simulink model "vipstripes"  (R2017b)
settings: Solver=FixedStepDiscrete  StartTime=0.0  StopTime=inf  RelTol=1e-3  EnableMultiTasking=on
model workspace (MATLAB code in the model file):
  | % Define image size and padded size.
  | imgSize = [120 160];
  | paddedSize = 2^ceil(log2(max(imgSize)));
  | 
  | % Load and initialize the data required by vipstripes demo.
  | cf = 0.65;
  | f = cf-0.04:0.005:cf+0.04;
  | f = repmat(f,[7,1]);
  | f = f(:);
  | ft.time=[];
  | ft.signals.values=f;
  | ft.signals.dimensions=1;
  | p = 0:0.5:3;
  | pt.time=[];
  | pt.signals.values=p';
  | pt.signals.dimensions= 1;
  | % FIR least-squares Bandstop filter designed using the FIRLS function.
  | % dfilt requires Signal Processing Toolbox license
  | % All frequency values are normalized to 1.
  | % N      = 30;    % Order
  | % Fpass1 = 0.51;  % First Passband Frequency
  | % Fstop1 = 0.6;   % First Stopband Frequency
  | % Fstop2 = 0.7;   % Second Stopband Frequency
  | % Fpass2 = 0.79;  % Second Passband Frequency
  | % Wpass1 = 1;     % First Passband Weight
  | % Wstop  = 1;     % Stopband Weight
  | % Wpass2 = 1;     % Second Passband Weight
  | % % Calculate the coefficients using the FIRLS function.
  | % Hd = dfilt.dffir(firls(N, [0 Fpass1 Fstop1 Fstop2 Fpass2 1], ...
  | %            [1 1 0 0 1 1], [Wpass1 Wstop Wpass2]));
  | %
  | % % Extract filter coefficients from the filter object
  | % b  = Hd.Numerator;
  | b = [ 0.0128   -0.0172    0.0010    0.0153   -0.0098 ...
  |       0.0002   -0.0149    0.0283    0.0129   -0.0852 ...
  |       0.0790    0.0478   -0.1639    0.1058    0.0897 ...
  |       0.8012    0.0897    0.1058   -0.1639    0.0478 ...
  |       0.0790   -0.0852    0.0129    0.0283   -0.0149 ...
  |       0.0002   -0.0098    0.0153    0.0010   -0.0172 ...
  |       0.0128 ];
  | % Convert the one-dimensional filter to 2-D using ftrans2 function from
  | % the Image Processing toolbox
  | h = ftrans2(b);
undefined symbols (not defined in the file or in its folder): gray
libraries: visiontransforms x2, visiontextngfix x2, visiongeotforms x2, visionutilities x1, visionfilter x1, vipmisc x1, dspvision x1
settings Model: FPTRunName=Active  ExtModeAutoUpdateStatusClock=off  Creator=The MathWorks, Inc.  LastModifiedBy=The MathWorks, Inc.
settings DataIOCC: LimitDataPoints=on  SaveFormat=Array  SaveOutput=off  SaveTime=off  SignalLoggingName=logsOut
settings OptimizationCC: ExpressionDepthLimit=2147483647  InitFltsAndDblsToZero=on  EfficientMapNaN2IntZero=off  LifeSpan=inf
settings DebuggingCC: SaveWithParameterizedLinksMsg=none  UnderspecifiedInitializationDetection=Classic  MergeDetectMultiDrivingBlocksExec=none  CheckExecutionContextPreStartOutputMsg=on  CheckExecutionContextRuntimeOutputMsg=on  SignalResolutionControl=TryResolveAllWithWarning  InheritedTsInSrcMsg=none  MultiTaskDSMMsg=warning  MultiTaskCondExecSysMsg=none  SigSpecEnsureSampleTimeMsg=none  ParameterPrecisionLossMsg=none  FcnCallInpInsideContextMsg=warning  AllowSymbolicDim=off  StateNameClashWarn=warning  SFUnexpectedBacktrackingDiag=warning  SFNoUnconditionalDefaultTransitionDiag=warning  SFExecutionAtInitializationDiag=none
settings HardwareCC: ProdBitPerPointer=32  ProdBitPerSizeT=32  ProdBitPerPtrDiffT=32  ProdLargestAtomicFloat=None  ProdIntDivRoundTo=Undefined  ProdEndianess=Unspecified  ProdWordSize=32  ProdHWDeviceType=32-bit Generic  TargetBitPerPointer=64  TargetBitPerSizeT=64  TargetBitPerPtrDiffT=64  TargetLongLongMode=on  TargetIntDivRoundTo=Zero  TargetEndianess=LittleEndian  TargetWordSize=64  TargetHWDeviceType=Generic->MATLAB Host Computer  ProdEqTarget=off
settings ModelReferenceCC: PropagateSignalLabelsOutOfModel=off
settings CodeAppCC: StateflowObjectComments=on
settings GRTTargetCC: TargetFcnLib=ansi_tfl_tmw.mat  TargetLangStandard=C89/C90 (ANSI)  GeneratePreprocessorConditionals=Disable all  CombineOutputUpdateFcns=off  GRTInterface=on
settings ConfigComp: CovMetricSettings=dw  CovHtmlReporting=on  CovSaveCumulativeToWorkspaceVar=on  CovSaveSingleToWorkspaceVar=on  CovExternalEMLEnable=off

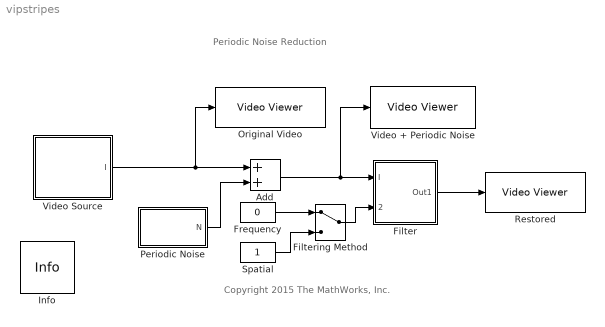
== system vipstripes ==
  note: Periodic Noise Reduction
  note: Copyright 2015 The MathWorks, Inc.
  Add : Sum
  Filter : Subsystem
  Filtering Method : ManualSwitch
  Frequency : Constant  Value=0
  Info : vipmisc/Info  SystemSampleTime=-1
      settings: SourceProductName=Computer Vision System Toolbox  SourceProductBaseCode=VP
  Original Video : VideoViewer  colormapValue=gray(256)  FigPos=[53 238 172 137]  trueSizedOnce=on
  Periodic Noise : Subsystem
  Restored : VideoViewer  colormapValue=gray(256)  FigPos=[50 623 172 127]  trueSizedOnce=on
  "Spatial " : Constant
  Video + Periodic Noise : VideoViewer  colormapValue=gray(256)  FigPos=[52 430 172 126]  trueSizedOnce=on
  Video Source : Subsystem
  wires:
  Video Source/1(I) -> Add/1, Original Video/1
  Periodic Noise/1(N) -> Add/2
  Add/1 -> Filter/1(I), Video + Periodic Noise/1
  Filter/1(Out1) -> Restored/1
  Frequency/1 -> Filtering Method/1
  "Spatial "/1 -> Filtering Method/2
  Filtering Method/1 -> Filter/2(Method)

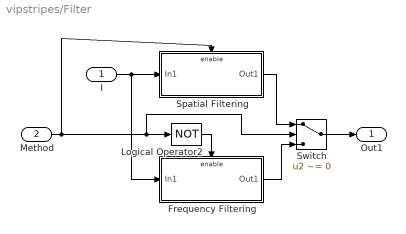
== system vipstripes/Filter ==
  I : Inport
  Method : Inport  Port=2
  Frequency Filtering : Subsystem  TreatAsAtomicUnit=on
  Logical Operator2 : Logic  Operator=NOT  AllPortsSameDT=off  OutDataTypeStr=boolean
  Spatial Filtering : Subsystem  TreatAsAtomicUnit=on
  Switch : Switch  Criteria=u2 ~= 0  ZeroCross=off
  Out1 : Outport
  wires:
  Logical Operator2/1 -> Frequency Filtering/Enable
  Method/1 -> Switch/2, Logical Operator2/1, Spatial Filtering/Enable
  Switch/1 -> Out1/1
  Frequency Filtering/1(Out1) -> Switch/3
  Spatial Filtering/1(Out1) -> Switch/1
  I/1 -> Frequency Filtering/1(In1), Spatial Filtering/1(In1)

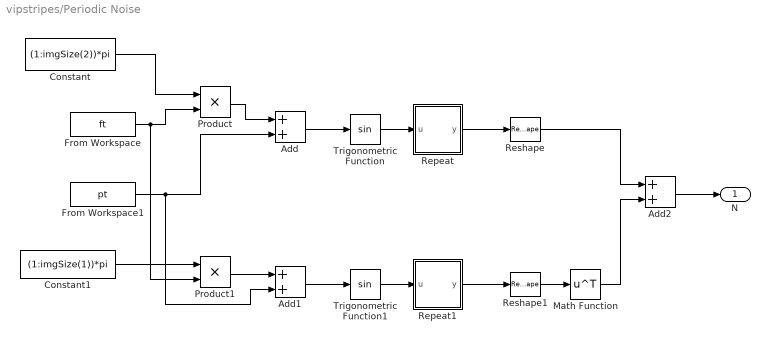
== system vipstripes/Periodic Noise ==
  Add : Sum
  Add1 : Sum
  Add2 : Sum
  Constant : Constant  Value=(1:imgSize(2))*pi
  Constant1 : Constant  Value=(1:imgSize(1))*pi
  From Workspace : FromWorkspace  VariableName=ft  Interpolate=off  OutputAfterFinalValue=Cyclic repetition
  From Workspace1 : FromWorkspace  VariableName=pt  Interpolate=off  OutputAfterFinalValue=Cyclic repetition
  Math Function : Math  Operator=transpose  SaturateOnIntegerOverflow=on
  Product : Product  RndMeth=Zero
  Product1 : Product  RndMeth=Zero
  Repeat : MATLAB Function  TreatAsAtomicUnit=on
  Repeat1 : MATLAB Function  TreatAsAtomicUnit=on
  Reshape : Reshape  OutputDimensionality=Customize  OutputDimensions=imgSize
  Reshape1 : Reshape  OutputDimensionality=Customize  OutputDimensions=fliplr(imgSize)
  Trigonometric Function : Trigonometry
  Trigonometric Function1 : Trigonometry
  N : Outport
  wires:
  Constant/1 -> Product/1
  From Workspace/1 -> Product/2, Product1/2
  Product/1 -> Add/1
  From Workspace1/1 -> Add/2, Add1/2
  Add/1 -> Trigonometric Function/1
  Trigonometric Function/1 -> Repeat/1(u)
  Repeat/1(y) -> Reshape/1
  Reshape/1 -> Add2/1
  Constant1/1 -> Product1/1
  Product1/1 -> Add1/1
  Add1/1 -> Trigonometric Function1/1
  Trigonometric Function1/1 -> Repeat1/1(u)
  Repeat1/1(y) -> Reshape1/1
  Reshape1/1 -> Math Function/1
  Math Function/1 -> Add2/2
  Add2/1 -> N/1

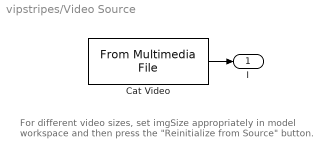
== system vipstripes/Video Source ==
  note: For different video sizes, set imgSize appropriately in model
      | workspace and then press the "Reinitialize from Source" button.
  Cat Video : dspvision/From Multimedia File  inputFilename=viptraffic.avi  loop=on  numPlays=inf  outputStreams=Video only  videoDataType=double  audioDataType=int16  inheritSampleTime=on  userDefinedSampleTime=1/30  noAudioOutput=off  isIntensityVideo=off  fourcc=Intensity  colorVideoFormat=Separate color signals  outputEOF=off  dataOrg=Column-major  audioFrameSize=1024  computeAudioFrameSize=off  outSamplingMode=Frame based
      settings: SourceProductBaseCode=VP
  I : Outport
  wires:
  Cat Video/1 -> I/1

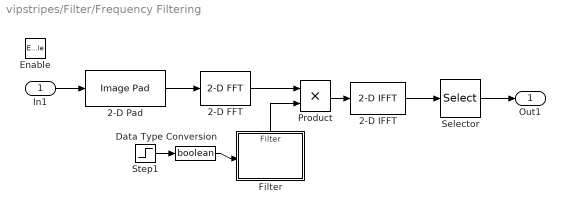
== system vipstripes/Filter/Frequency Filtering ==
  In1 : Inport
  Enable : EnablePort  PropagateVarSize=During execution
  2-D FFT : visiontransforms/2-D FFT  TableOpt=NEW  TableOptActive=Speed  BitRevOrder=off  SkipNorm=off  FFTImplementation=Auto  firstCoeffDataTypeStr=Inherit: Same word length as input  firstCoeffLastDataTypeStr=Inherit: Same word length as input  outputMin=[]  outputMax=[]  accumDataTypeStr=Inherit: Same as product output  accumLastDataTypeStr=Inherit: Same as product output  roundingMode=Floor  overflowMode=off
      settings: SourceProductName=Computer Vision System Toolbox  SourceProductBaseCode=VP
  2-D IFFT : visiontransforms/2-D IFFT  TableOpt=HYBRID  TableOptActive=Speed  BitRevOrder=off  cs_in=on  SkipNorm=on  FFTImplementation=Auto  firstCoeffDataTypeStr=Inherit: Same word length as input  firstCoeffLastDataTypeStr=Inherit: Same word length as input  outputMin=[]  outputMax=[]  accumDataTypeStr=Inherit: Same as product output  accumLastDataTypeStr=Inherit: Same as product output  roundingMode=Floor  overflowMode=off
      settings: SourceProductName=Computer Vision System Toolbox  SourceProductBaseCode=VP
  2-D Pad : visionutilities/Image Pad  method=Constant  valSrc=Specify via dialog  value=0  spec=Output size  rowDirection=Right  outRowsMode=User-specified  rowSize=2  outColSize=paddedSize  colDirection=Bottom  outColsMode=User-specified  colSize=[2 3]  outRowSize=paddedSize  trunc_flag=None
      settings: SourceProductName=Computer Vision System Toolbox  SourceProductBaseCode=VP
  Data Type Conversion : DataTypeConversion  OutDataTypeStr=boolean
  Filter : Subsystem  TreatAsAtomicUnit=on
  Product : Product  RndMeth=Zero
  Selector : Selector  NumberOfDimensions=2  InputPortWidth=3  IndexOptions=Index vector (dialog),Index vector (dialog)  Indices=[1:imgSize(1)],[1:imgSize(2)]  OutputSizes=1,1
  Step1 : Step  Time=eps  Before=1  After=0
  Out1 : Outport
  wires:
  In1/1 -> 2-D Pad/1
  Selector/1 -> Out1/1
  Step1/1 -> Data Type Conversion/1
  2-D IFFT/1 -> Selector/1
  2-D FFT/1 -> Product/1
  Product/1 -> 2-D IFFT/1
  2-D Pad/1 -> 2-D FFT/1
  Filter/1(Filter) -> Product/2
  Data Type Conversion/1 -> Filter/Enable

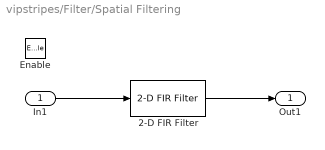
== system vipstripes/Filter/Spatial Filtering ==
  In1 : Inport
  Enable : EnablePort  PropagateVarSize=During execution
  2-D FIR Filter : visionfilter/2-D FIR Filter  separable=off  filtSrc=Specify via dialog  filterMtrx=h  verticalFilter=[4 0]  horizontalFilter=[4 0]  outSize=Same as input port I  padType=Circular  padSrc=Specify via dialog  padVal=0  method=Convolution  firstCoeffSignedness=Signed  firstCoeffDataTypeStr=Inherit: Same word length as input  firstCoeffLastDataTypeStr=Inherit: Same word length as input  firstCoeffMin=[]  firstCoeffMax=[]  outputSignedness=Auto  outputMin=[]  outputMax=[]  accumDataTypeStr=Inherit: Same as product output  accumLastDataTypeStr=Inherit: Same as product output  roundingMode=Floor  overflowMode=off
      settings: SourceProductName=Computer Vision System Toolbox  SourceProductBaseCode=VP
  Out1 : Outport
  wires:
  2-D FIR Filter/1 -> Out1/1
  In1/1 -> 2-D FIR Filter/1

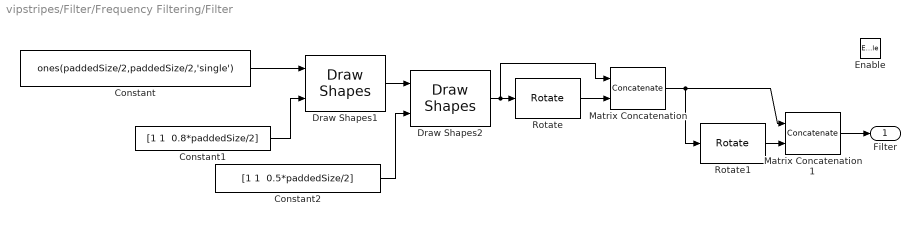
== system vipstripes/Filter/Frequency Filtering/Filter ==
  Enable : EnablePort  PropagateVarSize=During execution
  Constant : Constant  Value=ones(paddedSize/2,paddedSize/2,'single')
  Constant1 : Constant  Value="[1 1  0.8*paddedSize/2]"
  Constant2 : Constant  Value="[1 1  0.5*paddedSize/2]"
  Draw Shapes1 : visiontextngfix/Draw Shapes  shape=Circles  fill=on  lineWidth=1  fillClrSource=Specify via dialog  display=Black  intensity=200  color=[200 255 100]  opacity=1  viewport=Entire image  antialiasing=off  inType=Intensity  imagePorts=One multidimensional signal  prodOutputMode=Binary point scaling  prodOutputWordLength=32  prodOutputFracLength=14  memoryMode=Specify word length  memoryWordLength=16  memoryFracLength=15  roundingMode=Floor  overflowMode=off
      settings: SourceProductName=Computer Vision System Toolbox
  Draw Shapes2 : visiontextngfix/Draw Shapes  shape=Circles  fill=on  lineWidth=1  fillClrSource=Specify via dialog  display=White  intensity=200  color=[200 255 100]  opacity=1  viewport=Entire image  antialiasing=off  inType=Intensity  imagePorts=One multidimensional signal  prodOutputMode=Binary point scaling  prodOutputWordLength=32  prodOutputFracLength=14  memoryMode=Specify word length  memoryWordLength=16  memoryFracLength=15  roundingMode=Floor  overflowMode=off
      settings: SourceProductName=Computer Vision System Toolbox
  Matrix Concatenation : Concatenate  Mode=Multidimensional array  ConcatenateDimension=2
  Matrix Concatenation1 : Concatenate  Mode=Multidimensional array
  Rotate : visiongeotforms/Rotate  outSizeR=Same as input image  src_angle=Specify via dialog  unit_angle=Degrees  angle=-pi/2  maxAngle=pi  dispImage=Center  method=Trigonometric function  fillVal=0  interpMethod=Nearest neighbor  prodOutputMode=Binary point scaling  prodOutputWordLength=32  prodOutputFracLength=10  roundingMode=Nearest  overflowMode=on
      settings: SourceProductName=Computer Vision System Toolbox
  Rotate1 : visiongeotforms/Rotate  outSizeR=Same as input image  src_angle=Specify via dialog  unit_angle=Degrees  angle=pi  maxAngle=pi  dispImage=Center  method=Trigonometric function  fillVal=0  interpMethod=Nearest neighbor  prodOutputMode=Binary point scaling  prodOutputWordLength=32  prodOutputFracLength=10  roundingMode=Nearest  overflowMode=on
      settings: SourceProductName=Computer Vision System Toolbox
  Filter : Outport
  wires:
  Constant/1 -> Draw Shapes1/1
  Constant1/1 -> Draw Shapes1/2
  Draw Shapes1/1 -> Draw Shapes2/1
  Constant2/1 -> Draw Shapes2/2
  Draw Shapes2/1 -> Rotate/1, Matrix Concatenation/1
  Rotate/1 -> Matrix Concatenation/2
  Rotate1/1 -> Matrix Concatenation1/2
  Matrix Concatenation1/1 -> Filter/1
  Matrix Concatenation/1 -> Rotate1/1, Matrix Concatenation1/1

== matlab function vipstripes/Periodic Noise/Repeat1 ==
  data: u input; y output size=imgSize(1)*imgSize(2); imgSize parameter
function y = fcn(u, imgSize)
%#codegen

y = u ( kron(1:imgSize(1), ones(1,imgSize(2)) ) );

== matlab function vipstripes/Periodic Noise/Repeat ==
  data: u input; y output size=imgSize(1)*imgSize(2); imgSize parameter
function y = fcn(u, imgSize)
%#codegen

y = u ( kron(1:imgSize(2), ones(1,imgSize(1)) ) );
